simulink model "sim1_nonmininum"  (R2018a)
settings: Solver=VariableStepAuto  StartTime=0.0  StopTime=60  RelTol=1e-3
values from neighbouring files (symbols this model uses):
  A = [-dG(2:end)',[1;0]]    [ex1_liu.m]    (also in ex1_liu_geso.m)
  B = nG(2:end)'    [ex1_liu.m]    (also in ex1_liu_geso.m)
  K = [0 1]*inv(Mx)*PcA    [ex1_liu.m]    (also in ex1_liu_geso.m = place(A,B,[p1 p2]))
  kr = inv([1 0]*inv(eye(2)-A+B*K)*B)    [ex1_liu.m]    (also in ex1_liu_geso.m)
  Ts = 0.1    [ex1_liu.m]
libraries: cstblocks x4, simulink x1
settings Model: Creator=Bismark  LastModifiedBy=Bismark

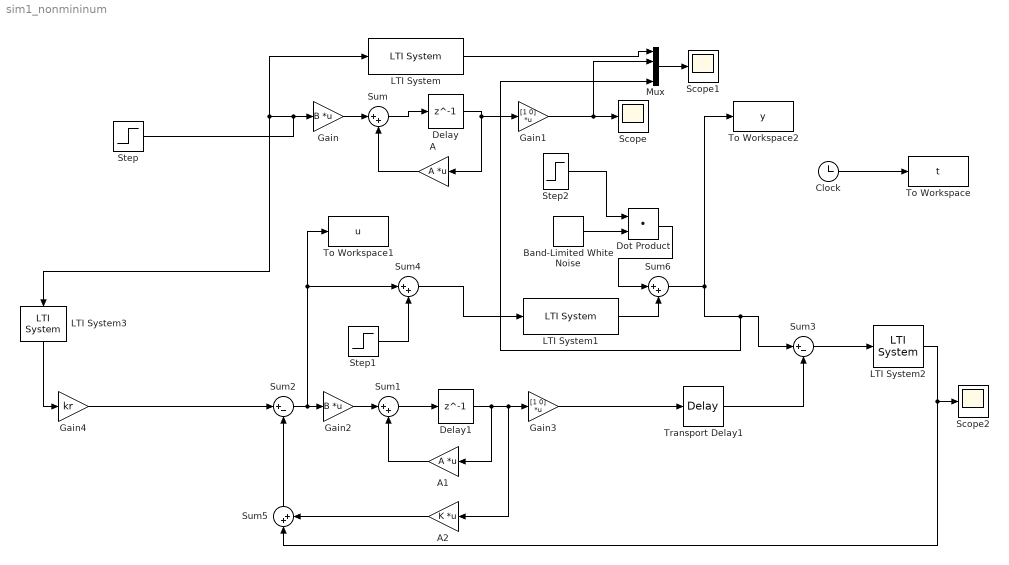
== system sim1_nonmininum ==
  A : Gain  Gain=A  Multiplication=Matrix(K*u) (u vector)
  A1 : Gain  Gain=A  Multiplication=Matrix(K*u) (u vector)
  A2 : Gain  Gain=K  Multiplication=Matrix(K*u) (u vector)
  Band-Limited White Noise : simulink/Sources/Band-Limited White Noise  Cov=[0.00001]  Ts=Ts  seed=[23341]
  Clock : Clock
  Delay : Delay  DelayLength=1  SampleTime=Ts
  Delay1 : Delay  DelayLength=1  SampleTime=Ts
  Dot Product : DotProduct  InputSameDT=on  OutDataTypeStr=Inherit: Inherit via internal rule
  Gain : Gain  Gain=B  Multiplication=Matrix(K*u) (u vector)
  Gain1 : Gain  Gain=[1 0]  Multiplication=Matrix(K*u)
  Gain2 : Gain  Gain=B  Multiplication=Matrix(K*u) (u vector)
  Gain3 : Gain  Gain=[1 0]  Multiplication=Matrix(K*u)
  Gain4 : Gain  Gain=kr
  LTI System : cstblocks/LTI System  sys=G  IC=[]
  LTI System1 : cstblocks/LTI System  sys=Pr  IC=[]
  LTI System2 : cstblocks/LTI System  sys=V  IC=[]
  LTI System3 : cstblocks/LTI System  sys=Fr  IC=[]
  Mux : Mux
  Scope : Scope
  Scope1 : Scope
  Scope2 : Scope
  Step : Step  Time=0  SampleTime=0
  Step1 : Step  Time=30  After=-1  SampleTime=Ts
  Step2 : Step  Time=55  SampleTime=0
  Sum{,1,4..6} (5 alike) : Sum  Inputs=|++
  Sum2 : Sum  Inputs=|+-
  Sum3 : Sum  Inputs=|+-
  To Workspace : ToWorkspace  VariableName=t  SampleTime=Ts
  To Workspace1 : ToWorkspace  VariableName=u  SampleTime=Ts
  To Workspace2 : ToWorkspace  VariableName=y  SampleTime=Ts
  Transport Delay1 : TransportDelay
  wires:
  Step/1 -> LTI System/1, LTI System3/1, Gain/1
  Gain/1 -> Sum/1
  A/1 -> Sum/2
  Sum/1 -> Delay/1
  Delay/1 -> A/1, Gain1/1
  Gain1/1 -> Mux/2, Scope/1
  LTI System/1 -> Mux/1
  Mux/1 -> Scope1/1
  Delay1/1 -> A1/1, A2/1, Gain3/1
  Sum1/1 -> Delay1/1
  Gain2/1 -> Sum1/1
  A1/1 -> Sum1/2
  Sum2/1 -> Sum4/1, To Workspace1/1, Gain2/1
  Gain4/1 -> Sum2/1
  Clock/1 -> To Workspace/1
  Gain3/1 -> Transport Delay1/1
  Transport Delay1/1 -> Sum3/2
  Sum4/1 -> LTI System1/1
  Step1/1 -> Sum4/2
  Sum6/1 -> Mux/4, Sum3/1, To Workspace2/1
  Sum5/1 -> Sum2/2
  A2/1 -> Sum5/2
  Sum3/1 -> LTI System2/1
  LTI System2/1 -> Scope2/1, Sum5/1
  LTI System3/1 -> Gain4/1
  Step2/1 -> Dot Product/1
  Band-Limited White Noise/1 -> Dot Product/2
  LTI System1/1 -> Sum6/2
  Dot Product/1 -> Sum6/1
